simulink model "Topic2_lspb"  (R2015a)
settings: Solver=ode45  StartTime=0.0  StopTime=10.0  RelTol=1e-3
undefined symbols (not defined in the file or in its folder): q, qd, qdd
libraries: roblocks x3, simulink x1
settings Model: Creator=Alexander Liao  LastModifiedBy=Alexander Liao

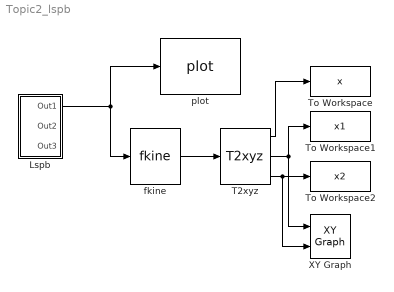
== system Topic2_lspb ==
  Lspb : Subsystem  mask{q0=[0,0,0,0,0,0,0,0], qf=[-0.4,-pi/2,-pi/2,pi/4,0,0,0,0], tmax=10, ts=0.05}
      mask init:
      | n = length(q0);
      | if length(q0) ~= length(qf) ,
      |  error('q0 and qf must be same length')
      | end
      | t=[0:100]'/100*tmax;
      | [q,qd,qdd] = mtraj(@lspb,q0,qf,t)
      mask Display:
      | port_label('output', 1, 'q')
      | port_label('output', 2, 'qd')
      | port_label('output', 3, 'qdd')
  T2xyz : roblocks/Transform Conversion/T2xyz
  To Workspace : ToWorkspace  VariableName=x  SampleTime=.05
      settings: Decimation=2  Save2DSignal=2-D array (concatenate along first dimension)
  To Workspace1 : ToWorkspace  VariableName=x1  SampleTime=.05
      settings: Decimation=2  Save2DSignal=2-D array (concatenate along first dimension)
  To Workspace2 : ToWorkspace  VariableName=x2  SampleTime=.05
      settings: Decimation=2  Save2DSignal=2-D array (concatenate along first dimension)
  XY Graph : simulink/Sinks/XY Graph  xmin=-1  xmax=1  ymin=-1  ymax=1  st=-1
  fkine : roblocks/Kinematics/fkine  robot=p560
  plot : roblocks/Robot Graphics/plot  robot=p560  fps=25  holdplot=on
  wires:
  fkine/1 -> T2xyz/1
  Lspb/1(Out1) -> plot/1, fkine/1
  T2xyz/3 -> XY Graph/2, To Workspace2/1
  T2xyz/1 -> To Workspace/1
  T2xyz/2 -> To Workspace1/1, XY Graph/1

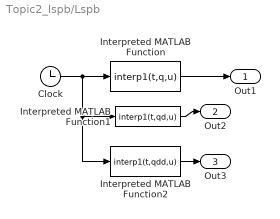
== system Topic2_lspb/Lspb ==
  Clock : Clock
  Interpreted MATLAB Function : MATLABFcn  MATLABFcn=interp1(t,q,u)  OutputDimensions=n
  Interpreted MATLAB Function1 : MATLABFcn  MATLABFcn=interp1(t,qd,u)  OutputDimensions=n
  Interpreted MATLAB Function2 : MATLABFcn  MATLABFcn=interp1(t,qdd,u)  OutputDimensions=n
  Out1 : Outport
  Out2 : Outport  Port=2
  Out3 : Outport  Port=3
  wires:
  Interpreted MATLAB Function/1 -> Out1/1
  Clock/1 -> Interpreted MATLAB Function2/1, Interpreted MATLAB Function1/1, Interpreted MATLAB Function/1
  Interpreted MATLAB Function2/1 -> Out3/1
  Interpreted MATLAB Function1/1 -> Out2/1
